simulink model "DetectStateMachine"  (R2016b)
settings: Solver=FixedStepDiscrete  StartTime=0.0  StopTime=inf  FixedStep=0.01  RelTol=1e-3
settings Model: Creator=chenjianhui  LastModifiedBy=chenjianhui
settings OptimizationCC: MaxStackSize=64
settings DebuggingCC: ParameterTunabilityLossMsg=error
settings HardwareCC: ProdBitPerLong=64  ProdHWDeviceType=Intel->x86-64 (Linux 64)
settings RTWCC: SystemTargetFile=ert.tlc  HardwareBoard=Robot Operating System (ROS)  TLCOptions="-aInlineSetEventsForThisBaseRateFcn=TLC_FALSE -aSuppressMultiTaskScheduler=TLC_FALSE  -aRateBasedStepFcn=0"  TemplateMakefile=ert_default_tmf  Description=Embedded Coder  GenerateReport=on  Toolchain=Catkin  IncludeHyperlinkInReport=on  LaunchReport=on  TargetLang=C++  GenerateTraceInfo=on  GenerateTraceReport=on  GenerateTraceReportSl=on  GenerateTraceReportSf=on  GenerateTraceReportEml=on
settings CodeAppCC: ForceParamTrailComments=on  IgnoreCustomStorageClasses=off  OperatorAnnotations=on  SimulinkDataObjDesc=on  SFDataObjDesc=on  MATLABFcnDesc=on  InsertBlockDesc=on  MATLABSourceComments=on

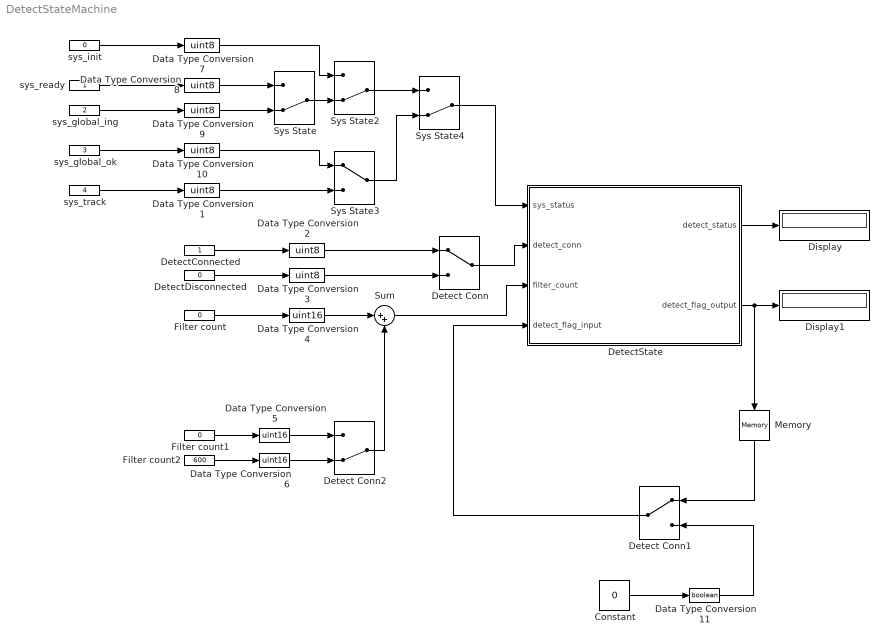
== system DetectStateMachine ==
  Constant : Constant  Value=0
  Data Type Conversion{1..3,7..10} (7 alike) : DataTypeConversion  OutDataTypeStr=uint8
  Data Type Conversion11 : DataTypeConversion  OutDataTypeStr=boolean
  Data Type Conversion4 : DataTypeConversion  OutDataTypeStr=uint16
  Data Type Conversion5 : DataTypeConversion  OutDataTypeStr=uint16
  Data Type Conversion6 : DataTypeConversion  OutDataTypeStr=uint16
  Detect Conn : ManualSwitch
  Detect Conn1 : ManualSwitch
  Detect Conn2 : ManualSwitch  CurrentSetting=0
  DetectConnected : Constant
  DetectDisconnected : Constant  Value=0
  DetectState : Stateflow chart  TreatAsAtomicUnit=on
  Display : Display
  Display1 : Display
  Filter count : Constant  Value=0
  Filter count1 : Constant  Value=0
  Filter count2 : Constant  Value=600
  Memory : Memory
  Sum : Sum  Inputs=|++
  Sys State : ManualSwitch  CurrentSetting=0
  Sys State2 : ManualSwitch  CurrentSetting=0
  Sys State3 : ManualSwitch
  Sys State4 : ManualSwitch  CurrentSetting=0
  sys_global_ing : Constant  Value=2
  sys_global_ok : Constant  Value=3
  sys_init : Constant  Value=0
  sys_ready : Constant
  sys_track : Constant  Value=4
  wires:
  DetectConnected/1 -> Data Type Conversion2/1
  DetectDisconnected/1 -> Data Type Conversion3/1
  Data Type Conversion2/1 -> Detect Conn/1
  Data Type Conversion3/1 -> Detect Conn/2
  Detect Conn/1 -> DetectState/2(detect_conn)
  Sys State/1 -> Sys State2/2
  sys_init/1 -> Data Type Conversion7/1
  sys_ready/1 -> Data Type Conversion8/1
  sys_global_ing/1 -> Data Type Conversion9/1
  Data Type Conversion1/1 -> Sys State3/2
  sys_global_ok/1 -> Data Type Conversion10/1
  Data Type Conversion7/1 -> Sys State2/1
  Data Type Conversion8/1 -> Sys State/1
  Data Type Conversion9/1 -> Sys State/2
  Data Type Conversion10/1 -> Sys State3/1
  sys_track/1 -> Data Type Conversion1/1
  Sys State2/1 -> Sys State4/1
  Sys State3/1 -> Sys State4/2
  Sys State4/1 -> DetectState/1(sys_status)
  DetectState/1(detect_status) -> Display/1
  Filter count/1 -> Data Type Conversion4/1
  DetectState/2(detect_flag_output) -> Display1/1, Memory/1
  Detect Conn1/1 -> DetectState/4(detect_flag_input)
  Filter count1/1 -> Data Type Conversion5/1
  Data Type Conversion4/1 -> Sum/1
  Sum/1 -> DetectState/3(filter_count)
  Detect Conn2/1 -> Sum/2
  Data Type Conversion5/1 -> Detect Conn2/1
  Filter count2/1 -> Data Type Conversion6/1
  Data Type Conversion6/1 -> Detect Conn2/2
  Constant/1 -> Data Type Conversion11/1
  Data Type Conversion11/1 -> Detect Conn1/2
  Memory/1 -> Detect Conn1/1

== stateflow chart DetectStateMachine/DetectState ==
  settings: updateMethod=DISCRETE  sampleTime=0.01
  state DetectFilter
    entry:cal_count = filter_count+counter_times;
    during:detect_status = 1;
  state DetectReady
    during:detect_status = 0;
  state DetectCal
    entry:detect_flag_output = true;
    during:detect_status = 1;
    exit:detect_flag_output = false;
  state DetectCalOK
    during:detect_status = 2;
  (default) -> DetectReady
  DetectReady -> DetectFilter : [detect_conn == 1 && ...
      | sys_status == 2]
  DetectFilter -> DetectReady [order 1] : [detect_conn == 0 || ...
      | sys_status != 2]
  DetectFilter -> DetectCal [order 2] : [filter_count >= cal_count]
  DetectCalOK -> DetectReady : [sys_status == 3 || ...
      | sys_status == 0 || ...
      | sys_status == 1 || ...
      | detect_conn == 0]
  DetectCal -> DetectCalOK : [detect_flag_input == false]
  data: sys_status input uint8; detect_conn input uint8; detect_status output uint8; counter_times parameter uint16; cal_count local uint16; filter_count input uint16; detect_flag_output output boolean =false; detect_flag_input input boolean
